simulink library "PoolIir"  (R2022b)
settings: Solver=VariableStepAuto  StartTime=0.0  StopTime=10.0  RelTol=1e-3
undefined symbols (not defined in the file or in its folder): Row
libraries: HandyTextFile x14, TuneVar x5, $bdroot x4, simulink x3, RTC x3, FeaturePath x2, TOP x2, AudioStats x1, CapturedConstLib x1
(part 1 of 2)
settings Model: Creator=sd49596  LastModifiedBy=fz1054048
settings SolverCC: AlgebraicLoopSolver=TrustRegion
settings DebuggingCC: UnconnectedInputMsg=warning  UnconnectedOutputMsg=warning  UnconnectedLineMsg=warning  SFMachineParentedDataDiag=warning  ArithmeticOperatorsInVariantConditions=warning
settings ModelReferenceCC: EnableRefExpFcnMdlSchedulingChecks=on
settings SFSimCC: CustomCodeUndefinedFunction=UseInterfaceOnly
settings RTWCC: DLArmComputeVersion=19.05

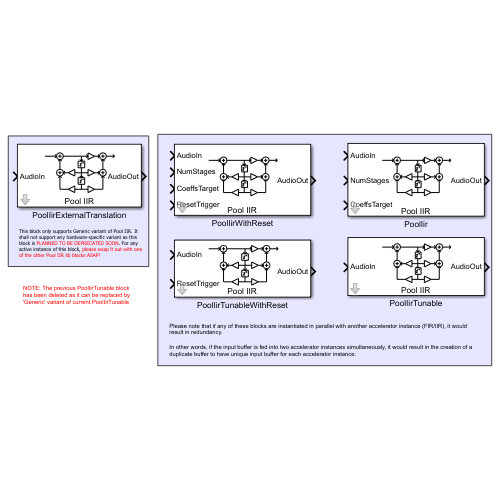
[thumbnail: Simulink's stored preview of the top-level diagram]
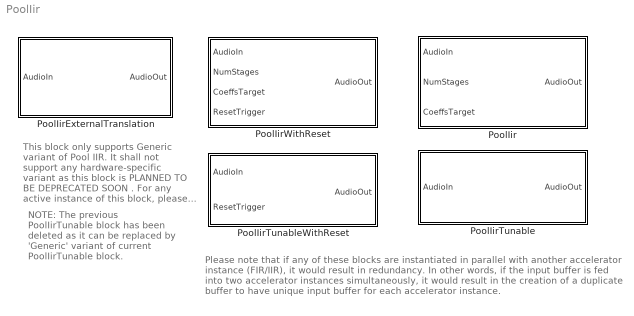
== system PoolIir ==
  note: NOTE: The previous PoolIirTunable block has been deleted as it can be replaced by 'Generic' variant of current PoolIirTunable block.
  note: This block only supports Generic variant of Pool IIR. It shall not support any hardware-specific variant as this block is PLANNED TO BE DEPRECATED SOON . For any active instance of this block, please swap it out with one of the other Pool IIR lib blocks ASAP!
  note: Please note that if any of these blocks are instantiated in parallel with another accelerator instance (FIR/IIR), it would result in redundancy.
      |
      | In other words, if the input buffer is fed into two accelerator instances simultaneously, it would result in the creation of a duplicate buffer to have unique input buffer for each accelerator instance.
  PoolIir : Subsystem  mask(Bose Pool IIR){Config=[]}
      mask prompts: Config "PoolIirConfig"
      mask help:
      | Pool IIR is a configurable multi-channel IIR filter that supports one or more channels. This block only supports the basic signal processing. The number of stages and coefficients need to be passed in in a format expected by the target. The Pool IIR block supports different implementations, which could be configured at build-time:
      |
      | (i)   Generic: IIR filter code not optimized for any processor
      | (ii)  SharcCore: IIR filters executing on core (uses pooliir.asm CRL)
      | (iii) SharcGulAccel: IIR filters executing on IIR hardware accelerator, offloading MIPS usage from core
      | (iv) SharcGxpAccel: IIR filters take advantage of additional accelerators available on GXP processor
      | (v)  Hexagon: TBD
      |
      | NOTE: When using Pool IIR for Sharc-plus based processors, the codeWorkMemory buffer and input buffer should always be mapped to L1 memory to optimize MIPS utilization and avoid audio artifacts.
      mask init:
      | blkh=gcbh;
      | Config=BTConfig.Assert(blkh,Config);
      | 
      | Config.Validate();
      | Config.DoMaskInit(blkh);
      mask Display: DrawPoolIirIcon;
  PoolIirExternalTranslation : Subsystem  InitFcn=warning('''%s'' block will soon be deprecated. Please replace all the active instances of ''PoolIirExternalTranslation'' with an appropriate BTC supported version of Pool IIR located within PoolIir.slx.', gcb);  mask{Config=[], FeatureName=filter}
      mask prompts: Config "PoolIirExternalTranslationConfig"; FeatureName "Feature path name:"
      mask init:
      | blkh=gcbh;
      | Config=BTConfig.Assert(blkh,Config);
      | 
      | BTConfig.InitSetFeatureIfPresent(blkh,'FeatureName');
      | Config.Validate();
      mask Callback Config: BTConfig.CallbackHideIfPresent(gcbh,{'FeatureName'});
      mask TypeOptions FeatureName: FeaturePath/FeatureName
      mask Display: DrawPoolIirIcon;
  PoolIirTunable : Subsystem  mask(Bose Pool IIR Tunable){FeatureName=PoolIirTunableConfig, Config=[]}
      mask prompts: FeatureName "Filter name/purpose"; Config "PoolIirTunableConfig"
      mask help:
      | Pool IIR Tunable is a configurable multi-channel IIR filter that supports one or more channels. This block offers flexibility of tuning the number of stages and coefficients. Different filter coefficients and number of stages (biquads) can be used for each channel filter. The Pool IIR Tunable block supports different implementations, which could be configured at build-time:
      |
      | (i)   Generic: IIR filter code not optimized for any processor
      | (ii)  SharcCore: IIR filters executing on core (uses pooliir.asm CRL)
      | (iii) SharcGulAccel: IIR filters executing on IIR hardware accelerator, offloading MIPS usage from core
      | (iv) SharcGxpAccel: IIR filters take advantage of additional accelerators available on GXP processor
      | (v)  Hexagon: TBD
      |
      | NOTE: When using Pool IIR for Sharc-plus based processors, the codeWorkMemory buffer and input buffer should always be mapped to L1 memory to optimize MIPS utilization and avoid audio artifacts.
      |
      | For more information, please see 'Help'.
      mask init:
      | blkh=gcbh;
      | Config=BTConfig.Assert(blkh,Config);
      | 
      | Config.Validate();
      | Config.DoMaskInit(blkh);
      mask Help:
      | <b>Input signals: </b>
      | AudioIn: input channels [frame size x number of channels]
      | 
      | <b>Output signals: </b>
      | AudioOut: output channels [frame size x number of channels]
      | 
      | <b>Mask parameters: </b>
      | PoolIirTunableConfig
      | Filter name/purpose
      mask TypeOptions FeatureName: PoolIirTunableWithReset/FeatureName
      mask Display: DrawPoolIirIcon;
  PoolIirTunableWithReset : Subsystem  mask(Bose Pool IIR Tunable With Reset){FeatureName=PoolIirTunableConfig, Config=[]}
      mask prompts: FeatureName "Filter name/purpose"; Config "PoolIirTunableWithResetConfig"
      mask help:
      | Pool IIR Tunable is a configurable multi-channel IIR filter that supports one or more channels. This block offers flexibility of tuning the number of stages and coefficients. Different filter coefficients and number of stages (biquads) can be used for each channel filter. The Pool IIR Tunable block supports different implementations, which could be configured at build-time:
      |
      | (i)   Generic: IIR filter code not optimized for any processor
      | (ii)  SharcCore: IIR filters executing on core (uses pooliir.asm CRL)
      | (iii) SharcGulAccel: IIR filters executing on IIR hardware accelerator, offloading MIPS usage from core
      | (iv) SharcGxpAccel: IIR filters take advantage of additional accelerators available on GXP processor
      | (v)  Hexagon: TBD
      |
      | NOTE: When using Pool IIR for Sharc-plus based processors, the codeWorkMemory buffer and input buffer should always be mapped to L1 memory to optimize MIPS utilization and avoid audio artifacts.
      |
      | For more information, please see 'Help'.
      mask init:
      | blkh=gcbh;
      | Config=BTConfig.Assert(blkh,Config);
      | 
      | BTConfig.InitSetFeatureIfPresent(blkh,'FeatureName');
      | Config.Validate();
      | Config.DoMaskInit(blkh);
      mask Help:
      | <b>Input signals: </b>
      | AudioIn: input channels [frame size x number of channels]
      | ResetTrigger: trigger to reset internal state buffer (usually preferred as a post RMDL step)
      | 
      | <b>Output signals: </b>
      | AudioOut: output channels [frame size x number of channels]
      | 
      | <b>Mask parameters: </b>
      | PoolIirTunableWithResetConfig
      | Filter name/purpose
      mask TypeOptions FeatureName: FeaturePath/FeatureName
      mask Callback Config: BTConfig.CallbackHideIfPresent(gcbh,{'FeatureName'});
      mask Display: DrawPoolIirIcon;
  PoolIirWithReset : Subsystem  mask(Bose Pool IIR With Reset){Config=[]}
      mask prompts: Config "PoolIirWithResetConfig"
      mask help:
      | Pool IIR is a configurable multi-channel IIR filter that supports one or more channels. This block only supports the basic signal processing. The number of stages and coefficients need to be passed in in a format expected by the target. The Pool IIR block supports different implementations, which could be configured at build-time:
      |
      | (i)   Generic: IIR filter code not optimized for any processor
      | (ii)  SharcCore: IIR filters executing on core (uses pooliir.asm CRL)
      | (iii) SharcGulAccel: IIR filters executing on IIR hardware accelerator, offloading MIPS usage from core
      | (iv) SharcGxpAccel: IIR filters take advantage of additional accelerators available on GXP processor
      | (v)  Hexagon: TBD
      |
      | NOTE: When using Pool IIR for Sharc-plus based processors, the codeWorkMemory buffer and input buffer should always be mapped to L1 memory to optimize MIPS utilization and avoid audio artifacts.
      mask init:
      | blkh=gcbh;
      | Config=BTConfig.Assert(blkh,Config);
      | 
      | Config.Validate();
      | Config.DoMaskInit(blkh);
      mask Display: DrawPoolIirIcon;

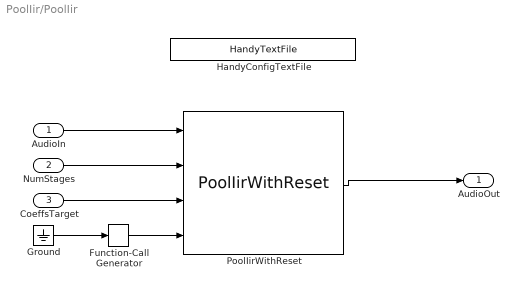
== system PoolIir/PoolIir ==
  AudioIn : Inport
  NumStages : Inport  Port=2
  CoeffsTarget : Inport  Port=3
  Function-Call Generator : simulink/Ports & Subsystems/Function-Call Generator  sample_time=1  numberOfIterations=1  DisallowWideOutput=off  ShowEnablePort=on
  Ground : Ground
  HandyConfigTextFile : HandyTextFile/HandyTextFile  TemplateSource=Config  FileSuffix=File  OpenDialogOnLoad=off  UseThisBlockName=off  AddGrandParentNamePrefix=off  TheDefaultText=% $(FILENAME) $(PREFIX) $(SUFFIX)  ShowInLibBrowser=on
      settings: SourceProductName=Bose Talaria
  PoolIirWithReset : $bdroot/PoolIirWithReset  Config=Config
  AudioOut : Outport
  wires:
  AudioIn/1 -> PoolIirWithReset/1
  PoolIirWithReset/1 -> AudioOut/1
  NumStages/1 -> PoolIirWithReset/2
  CoeffsTarget/1 -> PoolIirWithReset/3
  Function-Call Generator/1 -> PoolIirWithReset/4
  Ground/1 -> Function-Call Generator/1

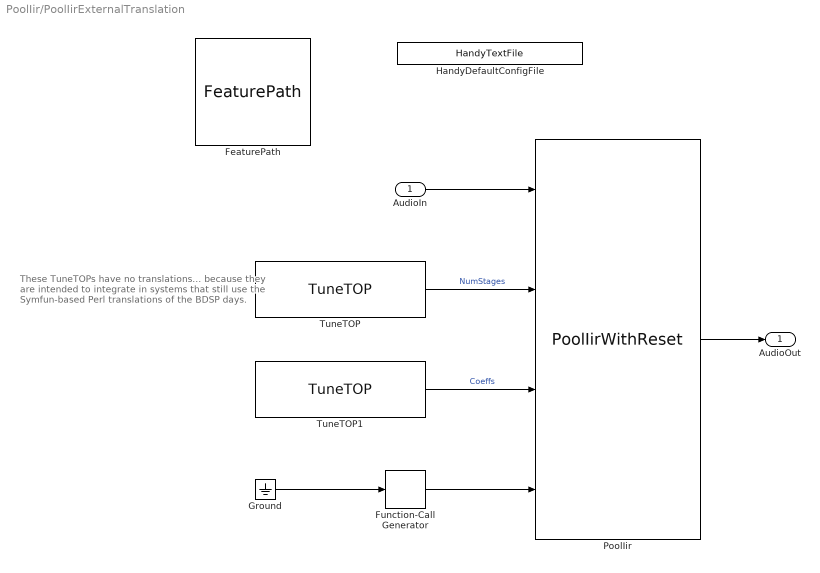
== system PoolIir/PoolIirExternalTranslation ==
  note: These TuneTOPs have no translations... because
      | they are intended to integrate in systems that still
      | use the Symfun-based Perl translations of the
      | BDSP days.
  AudioIn : Inport
  FeaturePath : FeaturePath/FeaturePath  FeatureName=filter  IsGroup=off  GroupNumber=-1  IsModule=off  TriggerInit=[-205 -51 -90 56]
      settings: SourceProductName=Bose Talaria
  Function-Call Generator : simulink/Ports & Subsystems/Function-Call Generator  sample_time=1  numberOfIterations=1  DisallowWideOutput=off  ShowEnablePort=on
  Ground : Ground
  HandyDefaultConfigFile : HandyTextFile/HandyTextFile  TemplateSource=Config  FileSuffix=Init  OpenDialogOnLoad=off  UseThisBlockName=off  AddGrandParentNamePrefix=off  TheDefaultText=|  ShowInLibBrowser=on
      | % $(FILENAME) Setup model parameters for each "Init" callback (e.g. update diagram)
      | sample_rate_in_hertz = 44100;
      | frame_size = 32;
      | sysin_channel_count = 2;
      settings: SourceProductName=Bose Talaria
  PoolIir : $bdroot/PoolIirWithReset  Config=Config.PoolIir
      settings: LibrarySourceBlock=PoolIir/PoolIir
  TuneTOP : TuneVar/TuneTOP  TriggerInit=[-145 172 25 228]  TopName=NumStages  TuneName=NumStages  DataTypeOut=single  TunabilityNumber=1  MinValue=[]  MaxValue=[]  BankNumber=0  PreOverlay=false  PostOverlay=false  UseSameName=on  MaskValue=Config.DefaultNumStages
      settings: SourceProductName=Bose Talaria
  TuneTOP1 : TuneVar/TuneTOP  TriggerInit=[-145 272 25 328]  TopName=Coeffs  TuneName=Coeffs  DataTypeOut=single  TunabilityNumber=1  MinValue=[]  MaxValue=[]  BankNumber=0  PreOverlay=false  PostOverlay=false  UseSameName=on  MaskValue=Config.DefaultSosCoefficients
      settings: SourceProductName=Bose Talaria
  AudioOut : Outport  VectorParamsAs1DForOutWhenUnconnected=off
  wires:
  TuneTOP1/1 -> PoolIir/3  "Coeffs"
  TuneTOP/1 -> PoolIir/2  "NumStages"
  AudioIn/1 -> PoolIir/1
  PoolIir/1 -> AudioOut/1
  Ground/1 -> Function-Call Generator/1
  Function-Call Generator/1 -> PoolIir/4

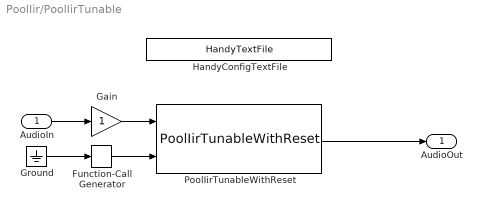
== system PoolIir/PoolIirTunable ==
  AudioIn : Inport
  Function-Call Generator : simulink/Ports & Subsystems/Function-Call Generator  sample_time=1  numberOfIterations=1  DisallowWideOutput=off  ShowEnablePort=on
  Gain : Gain
  Ground : Ground
  HandyConfigTextFile : HandyTextFile/HandyTextFile  TemplateSource=Config  FileSuffix=File  OpenDialogOnLoad=off  UseThisBlockName=off  AddGrandParentNamePrefix=off  TheDefaultText=% $(FILENAME) $(PREFIX) $(SUFFIX)  ShowInLibBrowser=on
      settings: SourceProductName=Bose Talaria
  PoolIirTunableWithReset : $bdroot/PoolIirTunableWithReset  FeatureName=PoolIirTunableConfig  Config=Config
  AudioOut : Outport
  wires:
  AudioIn/1 -> Gain/1
  PoolIirTunableWithReset/1 -> AudioOut/1
  Function-Call Generator/1 -> PoolIirTunableWithReset/2
  Ground/1 -> Function-Call Generator/1
  Gain/1 -> PoolIirTunableWithReset/1

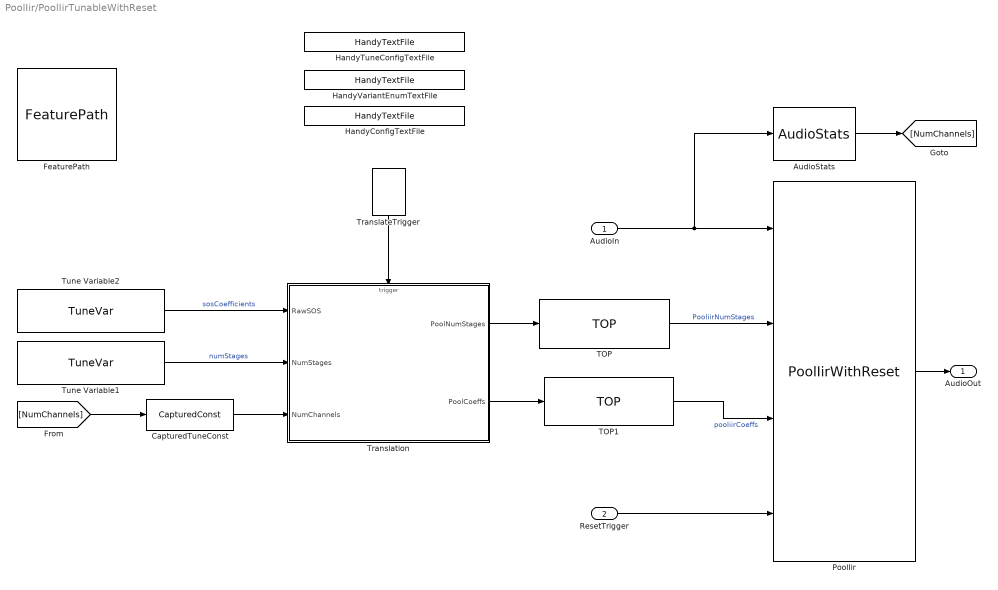
== system PoolIir/PoolIirTunableWithReset ==
  AudioIn : Inport
  ResetTrigger : Inport  Port=2
  AudioStats : AudioStats/AudioStats  DoSampleRate=off  TypeSampleRate=Inherit: auto  DoCallRate=off  TypeCallRate=Inherit: auto  DoFrameSize=off  TypeFrameSize=Inherit: auto  DoChannelCount=on  TypeChannelCount=int32  DoTaskRateFactor=off  TypeTaskRateFactor=Inherit: auto  MacroNameRoot=AUDIO  MacroNameRootEval='AUDIO'  IsMacroNameEval=off  MacroSampleRate=off  MacroCallRate=off  MacroFrameSize=off  MacroChannelCount=off  MacroTaskRateFactor=off  MacroTaskId=off  ValidateSampleRate=off  ValueSampleRate=[]  ValidateCallRate=off  ValueCallRate=[]  ValidateFrameSize=off  ValueFrameSize=[]  ValidateChannelCount=off  ValueChannelCount=[]  ValidateTaskRateFactor=off  ValueTaskRateFactor=[]
      settings: SourceProductName=Bose Talaria
  CapturedTuneConst : CapturedConstLib/CapturedConst  TriggerInit=[-600 302 -500 338]  Role=Automatic
      settings: SourceProductName=Bose Talaria
  FeaturePath : FeaturePath/FeaturePath  FeatureName=PoolIirTunableConfig  IsGroup=off  GroupNumber=-1  IsModule=off  TriggerInit=[-750 -81 -635 26]
      settings: SourceProductName=Bose Talaria
  HandyConfigTextFile : HandyTextFile/HandyTextFile  TemplateSource=Config  FileSuffix=File  OpenDialogOnLoad=off  UseThisBlockName=off  AddGrandParentNamePrefix=off  TheDefaultText=% $(FILENAME) $(PREFIX) $(SUFFIX)  ShowInLibBrowser=on
      settings: SourceProductName=Bose Talaria
  HandyTuneConfigTextFile : HandyTextFile/HandyTextFile  TemplateSource=TuneConfig  FileSuffix=File  OpenDialogOnLoad=off  UseThisBlockName=off  AddGrandParentNamePrefix=off  TheDefaultText=% $(FILENAME) $(PREFIX) $(SUFFIX)  ShowInLibBrowser=on
      settings: SourceProductName=Bose Talaria
  HandyVariantEnumTextFile : HandyTextFile/HandyTextFile  TemplateSource=VariantEnum  FileSuffix=File  OpenDialogOnLoad=off  UseThisBlockName=off  AddGrandParentNamePrefix=off  TheDefaultText=% $(FILENAME) $(PREFIX) $(SUFFIX)  ShowInLibBrowser=on
      settings: SourceProductName=Bose Talaria
  PoolIir : $bdroot/PoolIirWithReset  Config=Config
  TOP : TOP/TOP  TriggerInit=[-145 187 5 243]  TopName=PooliirNumStages  DataTypeOut=uint32  BankNumber=0  PreOverlay=false  PostOverlay=Config.BreedObj.PostOverlayRequired  CompatibilityString=Config.Breed  Role=Automatic
      settings: SourceProductName=Bose Talaria
  TOP1 : TOP/TOP  TriggerInit=[-140 277 10 333]  TopName=pooliirCoeffs  DataTypeOut=single  BankNumber=0  PreOverlay=false  PostOverlay=Config.BreedObj.PostOverlayRequired  CompatibilityString=Config.Breed  Role=Automatic
      settings: SourceProductName=Bose Talaria
  TranslateTrigger : TuneVar/TranslateTrigger  TriggerInit=[-339 35 -301 90]
      settings: SourceProductName=Bose Talaria
  Translation : MATLAB Function  TreatAsAtomicUnit=on  mask{MaxNumStages=Config.MaxNumStages, Breed=Config.Breed}
  Tune Variable1 : TuneVar/TuneVar  TuneName=numStages  SpecifyMaxSize=off  VariableDim=1 (Row)  MaxSize=[1 1]  TunabilityNumber=1  MinValue=[]  MaxValue=[]  TriggerInit=[-750 235 -580 285]  MaskValue=Config.TuneVarNumStages
      settings: SourceProductName=Bose Talaria
  Tune Variable2 : TuneVar/TuneVar  TuneName=sosCoefficients  SpecifyMaxSize=on  VariableDim=1 (Row)  MaxSize=[Config.MaxNumStages 6]  TunabilityNumber=1  MinValue=[]  MaxValue=[]  TriggerInit=[-750 175 -580 225]  MaskValue=Config.TuneVarSosCoefficients
      settings: SourceProductName=Bose Talaria
  AudioOut : Outport  VectorParamsAs1DForOutWhenUnconnected=off
  wires:
  AudioIn/1 -> AudioStats/1, PoolIir/1
  TOP/1 -> PoolIir/2  "PooliirNumStages"
  TOP1/1 -> PoolIir/3  "pooliirCoeffs"
  PoolIir/1 -> AudioOut/1
  TranslateTrigger/1 -> Translation/Trigger
  Tune Variable2/1 -> Translation/1(RawSOS)  "sosCoefficients"
  Translation/2(PoolCoeffs) -> TOP1/1
  Translation/1(PoolNumStages) -> TOP/1
  Tune Variable1/1 -> Translation/2(NumStages)  "numStages"
  ResetTrigger/1 -> PoolIir/4
  AudioStats/1 -> [NumChannels]
  [NumChannels] -> CapturedTuneConst/1
  CapturedTuneConst/1 -> Translation/3(NumChannels)

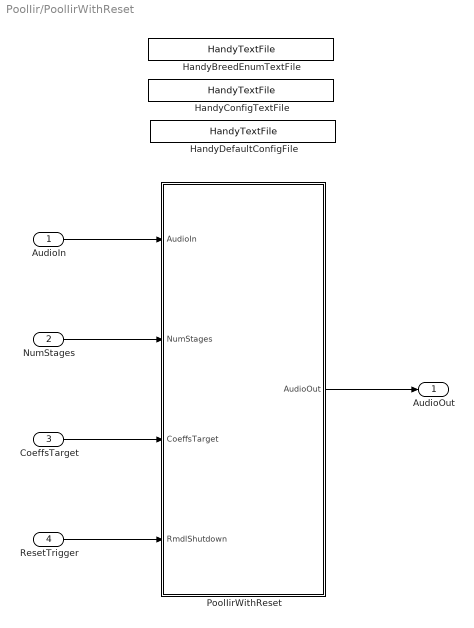
== system PoolIir/PoolIirWithReset ==
  AudioIn : Inport
  NumStages : Inport  Port=2
  CoeffsTarget : Inport  Port=3
  ResetTrigger : Inport  Port=4
  HandyBreedEnumTextFile : HandyTextFile/HandyTextFile  TemplateSource=<dialog fields>  FileSuffix=BreedEnum  OpenDialogOnLoad=off  UseThisBlockName=off  AddGrandParentNamePrefix=off  TheDefaultText=% $(FILENAME) $(PREFIX) $(SUFFIX)  ShowInLibBrowser=on
      settings: SourceProductName=Bose Talaria
  HandyConfigTextFile : HandyTextFile/HandyTextFile  TemplateSource=Config  FileSuffix=File  OpenDialogOnLoad=off  UseThisBlockName=off  AddGrandParentNamePrefix=off  TheDefaultText=% $(FILENAME) $(PREFIX) $(SUFFIX)  ShowInLibBrowser=on
      settings: SourceProductName=Bose Talaria
  HandyDefaultConfigFile : HandyTextFile/HandyTextFile  TemplateSource=Config  FileSuffix=Init  OpenDialogOnLoad=off  UseThisBlockName=off  AddGrandParentNamePrefix=off  TheDefaultText=|  ShowInLibBrowser=on
      | % $(FILENAME) Setup model parameters for each "Init" callback (e.g. update diagram)
      | sample_rate_in_hertz = 44100;
      | frame_size = 32;
      | sysin_channel_count = 2;
      settings: SourceProductName=Bose Talaria
  PoolIirWithReset : Subsystem  Variant=on
  AudioOut : Outport  VectorParamsAs1DForOutWhenUnconnected=off
  wires:
  AudioIn/1 -> PoolIirWithReset/1(AudioIn)
  ResetTrigger/1 -> PoolIirWithReset/4(RmdlShutdown)
  NumStages/1 -> PoolIirWithReset/2(NumStages)
  CoeffsTarget/1 -> PoolIirWithReset/3(CoeffsTarget)
  PoolIirWithReset/1(AudioOut) -> AudioOut/1

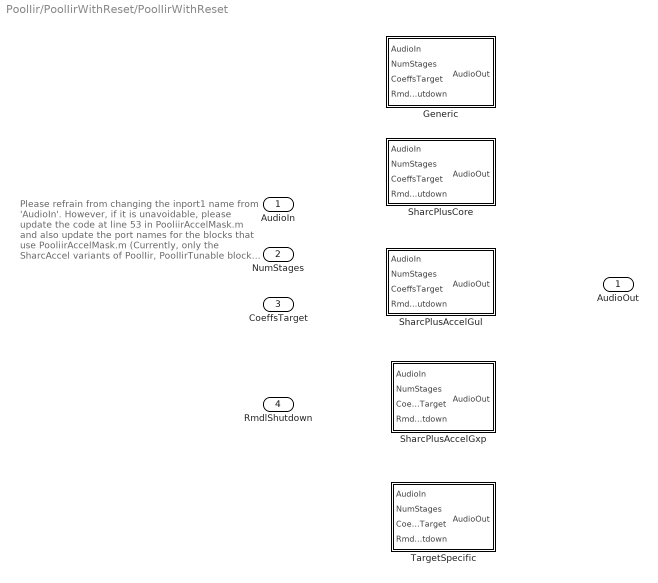
== system PoolIir/PoolIirWithReset/PoolIirWithReset ==
  note: Please refrain from changing the inport1 name from 'AudioIn'. However, if it is unavoidable, please update the code at line 53 in PooliirAccelMask.m and also update the port names for the blocks that use PooliirAccelMask.m (Currently, only the SharcAccel variants of PoolIir, PoolIirTunable block and PooliirAccelRmdl block uses that.)
  AudioIn : Inport
  NumStages : Inport  Port=2
  CoeffsTarget : Inport  Port=3
  RmdlShutdown : Inport  Port=4
  Generic : Subsystem  VariantControl=(default)
  SharcPlusAccelGul : Subsystem  VariantControl=Config.Breed == AsdHwEnum.SharcPlusAccelGul
  SharcPlusAccelGxp : Subsystem  VariantControl=Config.Breed == AsdHwEnum.SharcPlusAccelGxp
  SharcPlusCore : Subsystem  VariantControl=Config.Breed == AsdHwEnum.SharcPlusCore
  TargetSpecific : Subsystem  VariantControl=(Config.Breed == AsdHwEnum.Hexagon) || (Config.Breed == AsdHwEnum.ArmNeonV7V8)
  AudioOut : Outport

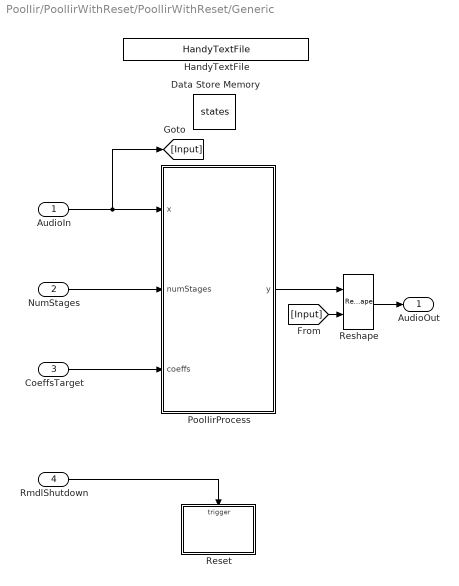
== system PoolIir/PoolIirWithReset/PoolIirWithReset/Generic ==
  AudioIn : Inport
  NumStages : Inport  Port=2
  CoeffsTarget : Inport  Port=3
  RmdlShutdown : Inport  Port=4
  Data Store Memory : DataStoreMemory  DataStoreName=states  InitialValue=Config.BreedObj.CodeWorkMemoryInitVal  ShowAdditionalParam=off  OutDataTypeStr=single
  HandyTextFile : HandyTextFile/HandyTextFile  TemplateSource=<dialog fields>  FileSuffix=BreedEnum  OpenDialogOnLoad=off  UseThisBlockName=off  AddGrandParentNamePrefix=on  TheDefaultText=% $(FILENAME) $(PREFIX) $(SUFFIX)  ShowInLibBrowser=on
      settings: SourceProductName=Bose Talaria
  PoolIirProcess : MATLAB Function  TreatAsAtomicUnit=on
  Reset : MATLAB Function  TreatAsAtomicUnit=on
  Reshape : Reshape  OutputDimensionality=Derive from reference input port
  AudioOut : Outport  VectorParamsAs1DForOutWhenUnconnected=off
  wires:
  RmdlShutdown/1 -> Reset/Trigger
  CoeffsTarget/1 -> PoolIirProcess/3(coeffs)
  NumStages/1 -> PoolIirProcess/2(numStages)
  Reshape/1 -> AudioOut/1
  AudioIn/1 -> [Input], PoolIirProcess/1(x)
  PoolIirProcess/1(y) -> Reshape/1
  [Input] -> Reshape/2

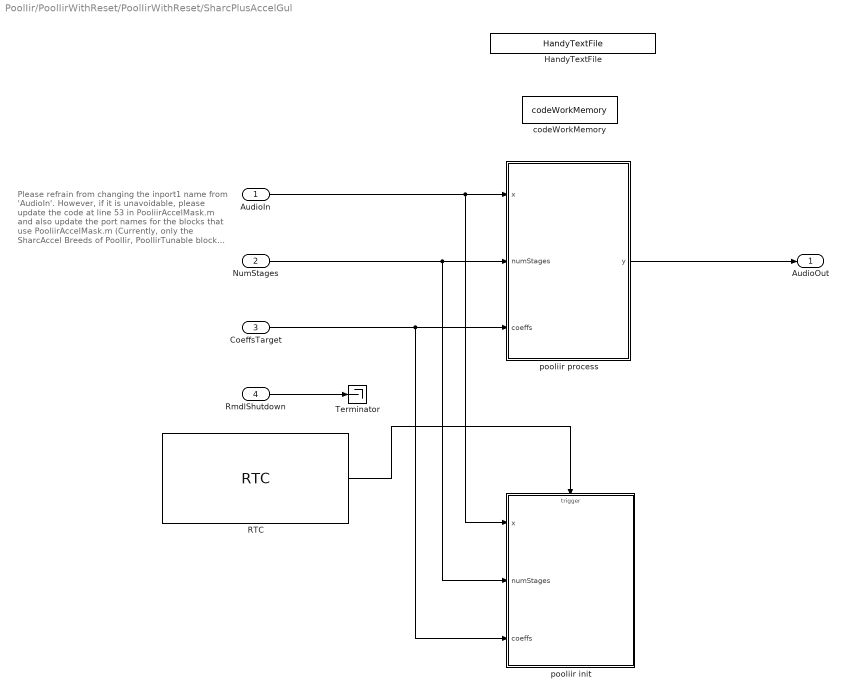
== system PoolIir/PoolIirWithReset/PoolIirWithReset/SharcPlusAccelGul ==
  note: Please refrain from changing the inport1 name from 'AudioIn'. However, if it is unavoidable, please update the code at line 53 in PooliirAccelMask.m and also update the port names for the blocks that use PooliirAccelMask.m (Currently, only the SharcAccel Breeds of PoolIir, PoolIirTunable block and PooliirAccelRmdl block uses that.)
  AudioIn : Inport
  NumStages : Inport  Port=2
  CoeffsTarget : Inport  Port=3
  RmdlShutdown : Inport  Port=4
  HandyTextFile : HandyTextFile/HandyTextFile  TemplateSource=<dialog fields>  FileSuffix=BreedEnum  OpenDialogOnLoad=off  UseThisBlockName=off  AddGrandParentNamePrefix=on  TheDefaultText=% $(FILENAME) $(PREFIX) $(SUFFIX)  ShowInLibBrowser=on
      settings: SourceProductName=Bose Talaria
  RTC : RTC/RTC  REQ_Priority=RTC_Mask.NormalPriority  RequestAtInit=on  EnableRequest=on  REQElemType1=uint32  REQElemWidth1=1  REQElemInitial1=[]  REQElemType2=uint32  REQElemWidth2=1  REQElemInitial2=[]  REQElemType3=uint32  REQElemWidth3=1  REQElemInitial3=[]  REQElemType4=uint32  REQElemWidth4=1  REQElemInitial4=[]  REQElemType5=uint32  REQElemWidth5=1  REQElemInitial5=[]  REQElemType6=uint32  REQElemWidth6=1  REQElemInitial6=[]  REQElemType7=uint32  REQElemWidth7=1  REQElemInitial7=[]  REQElemType8=uint32  REQElemWidth8=1  REQElemInitial8=[]  REQElemType9=uint32  REQElemWidth9=1  REQElemInitial9=[]  REQElemType10=uint32  REQElemWidth10=1  REQElemInitial10=[]  EnableResponse=off  EnableRSP_StatusIn=off  RSPElemType1=uint32  RSPElemWidth1=1  RSPElemType2=uint32  RSPElemWidth2=1  RSPElemType3=uint32  RSPElemWidth3=1  RSPElemType4=uint32  RSPElemWidth4=1  RSPElemType5=uint32  RSPElemWidth5=1  RSPElemType6=uint32  RSPElemWidth6=1  RSPElemType7=uint32  RSPElemWidth7=1  RSPElemType8=uint32  RSPElemWidth8=1  RSPElemType9=uint32  RSPElemWidth9=1  RSPElemType10=uint32  RSPElemWidth10=1  EnableNotification=off  EnableNTF_PrepTrig=off  NTFElemType1=uint32  NTFElemWidth1=1  NTFElemType2=uint32  NTFElemWidth2=1  NTFElemType3=uint32  NTFElemWidth3=1  NTFElemType4=uint32  NTFElemWidth4=1  NTFElemType5=uint32  NTFElemWidth5=1  NTFElemType6=uint32  NTFElemWidth6=1  NTFElemType7=uint32  NTFElemWidth7=1  NTFElemType8=uint32  NTFElemWidth8=1  NTFElemType9=uint32  NTFElemWidth9=1  NTFElemType10=uint32  NTFElemWidth10=1  MaskMessageName=PoolIirSharcPlusAccelGulInitReset
      settings: SourceProductName=Bose Talaria
  Terminator : Terminator
  codeWorkMemory : DataStoreMemory  DataStoreName=codeWorkMemory  WriteAfterWriteMsg=warning  InitialValue=Config.BreedObj.CodeWorkMemoryInitVal  ShowAdditionalParam=off  OutDataTypeStr=single
  pooliir init : MATLAB Function  TreatAsAtomicUnit=on  RTWFcnName=foo
  pooliir process : MATLAB Function  TreatAsAtomicUnit=on
  AudioOut : Outport  VectorParamsAs1DForOutWhenUnconnected=off
  wires:
  RmdlShutdown/1 -> Terminator/1
  CoeffsTarget/1 -> pooliir process/3(coeffs), pooliir init/3(coeffs)
  AudioIn/1 -> pooliir init/1(x), pooliir process/1(x)
  NumStages/1 -> pooliir process/2(numStages), pooliir init/2(numStages)
  RTC/1 -> pooliir init/Trigger
  pooliir process/1(y) -> AudioOut/1

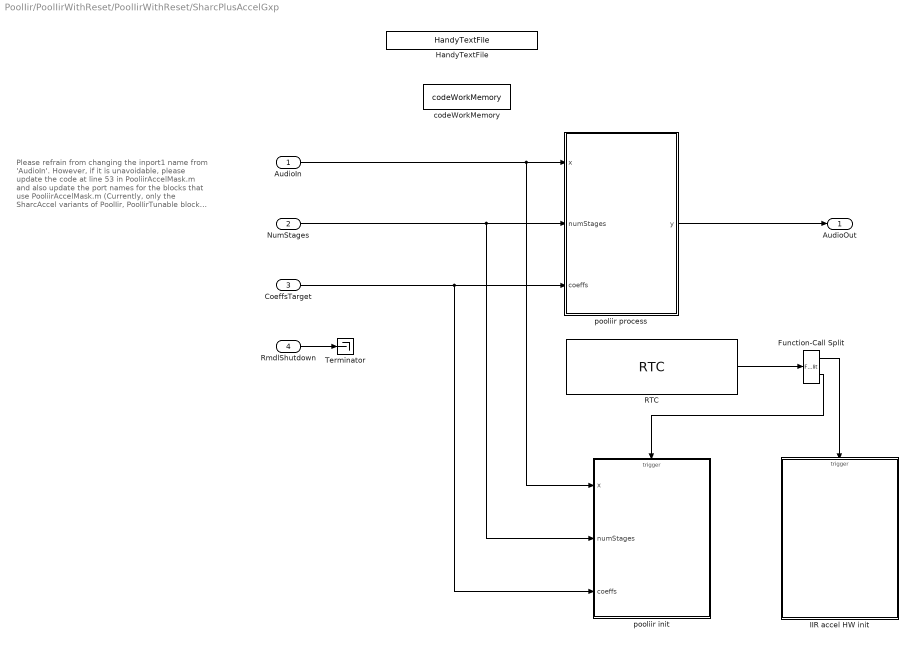
== system PoolIir/PoolIirWithReset/PoolIirWithReset/SharcPlusAccelGxp ==
  note: Please refrain from changing the inport1 name from 'AudioIn'. However, if it is unavoidable, please update the code at line 53 in PooliirAccelMask.m and also update the port names for the blocks that use PooliirAccelMask.m (Currently, only the SharcAccel variants of PoolIir, PoolIirTunable block and PooliirAccelRmdl block uses that.)
  AudioIn : Inport
  NumStages : Inport  Port=2
  CoeffsTarget : Inport  Port=3
  RmdlShutdown : Inport  Port=4
  Function-Call Split : FunctionCallSplit  NumOutputPorts=2  OutputPortLayout=default
  HandyTextFile : HandyTextFile/HandyTextFile  TemplateSource=<dialog fields>  FileSuffix=BreedEnum  OpenDialogOnLoad=off  UseThisBlockName=off  AddGrandParentNamePrefix=on  TheDefaultText=% $(FILENAME) $(PREFIX) $(SUFFIX)  ShowInLibBrowser=on
      settings: SourceProductName=Bose Talaria
  IIR accel HW init : MATLAB Function  TreatAsAtomicUnit=on  RTWFcnName=foo  mask{CoreId=Config.BreedObj.CoreId, AccelDeviceId=Config.BreedObj.AccelDeviceId}
  RTC : RTC/RTC  REQ_Priority=RTC_Mask.NormalPriority  RequestAtInit=on  EnableRequest=on  REQElemType1=uint32  REQElemWidth1=1  REQElemInitial1=[]  REQElemType2=uint32  REQElemWidth2=1  REQElemInitial2=[]  REQElemType3=uint32  REQElemWidth3=1  REQElemInitial3=[]  REQElemType4=uint32  REQElemWidth4=1  REQElemInitial4=[]  REQElemType5=uint32  REQElemWidth5=1  REQElemInitial5=[]  REQElemType6=uint32  REQElemWidth6=1  REQElemInitial6=[]  REQElemType7=uint32  REQElemWidth7=1  REQElemInitial7=[]  REQElemType8=uint32  REQElemWidth8=1  REQElemInitial8=[]  REQElemType9=uint32  REQElemWidth9=1  REQElemInitial9=[]  REQElemType10=uint32  REQElemWidth10=1  REQElemInitial10=[]  EnableResponse=off  EnableRSP_StatusIn=off  RSPElemType1=uint32  RSPElemWidth1=1  RSPElemType2=uint32  RSPElemWidth2=1  RSPElemType3=uint32  RSPElemWidth3=1  RSPElemType4=uint32  RSPElemWidth4=1  RSPElemType5=uint32  RSPElemWidth5=1  RSPElemType6=uint32  RSPElemWidth6=1  RSPElemType7=uint32  RSPElemWidth7=1  RSPElemType8=uint32  RSPElemWidth8=1  RSPElemType9=uint32  RSPElemWidth9=1  RSPElemType10=uint32  RSPElemWidth10=1  EnableNotification=off  EnableNTF_PrepTrig=off  NTFElemType1=uint32  NTFElemWidth1=1  NTFElemType2=uint32  NTFElemWidth2=1  NTFElemType3=uint32  NTFElemWidth3=1  NTFElemType4=uint32  NTFElemWidth4=1  NTFElemType5=uint32  NTFElemWidth5=1  NTFElemType6=uint32  NTFElemWidth6=1  NTFElemType7=uint32  NTFElemWidth7=1  NTFElemType8=uint32  NTFElemWidth8=1  NTFElemType9=uint32  NTFElemWidth9=1  NTFElemType10=uint32  NTFElemWidth10=1  MaskMessageName=PoolIirSharcPlusAccelGxpInitReset
      settings: SourceProductName=Bose Talaria
  Terminator : Terminator
  codeWorkMemory : DataStoreMemory  DataStoreName=codeWorkMemory  WriteAfterWriteMsg=warning  InitialValue=Config.BreedObj.CodeWorkMemoryInitVal  ShowAdditionalParam=off  OutDataTypeStr=single
  pooliir init : MATLAB Function  TreatAsAtomicUnit=on  RTWFcnName=foo  mask{AccelDeviceId=Config.BreedObj.AccelDeviceId}
  pooliir process : MATLAB Function  TreatAsAtomicUnit=on
  AudioOut : Outport
  wires:
  RmdlShutdown/1 -> Terminator/1
  CoeffsTarget/1 -> pooliir init/3(coeffs), pooliir process/3(coeffs)
  pooliir process/1(y) -> AudioOut/1
  AudioIn/1 -> pooliir init/1(x), pooliir process/1(x)
  NumStages/1 -> pooliir init/2(numStages), pooliir process/2(numStages)
  RTC/1 -> Function-Call Split/1
  Function-Call Split/2 -> pooliir init/Trigger
  Function-Call Split/1 -> IIR accel HW init/Trigger

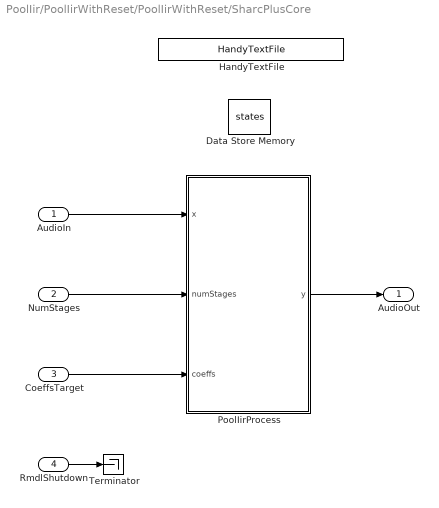
== system PoolIir/PoolIirWithReset/PoolIirWithReset/SharcPlusCore ==
  AudioIn : Inport
  NumStages : Inport  Port=2
  CoeffsTarget : Inport  Port=3
  RmdlShutdown : Inport  Port=4
  Data Store Memory : DataStoreMemory  DataStoreName=states  InitialValue=Config.BreedObj.CodeWorkMemoryInitVal  ShowAdditionalParam=off  OutDataTypeStr=single
  HandyTextFile : HandyTextFile/HandyTextFile  TemplateSource=<dialog fields>  FileSuffix=BreedConfig  OpenDialogOnLoad=off  UseThisBlockName=off  AddGrandParentNamePrefix=on  TheDefaultText=% $(FILENAME) $(PREFIX) $(SUFFIX)  ShowInLibBrowser=on
      settings: SourceProductName=Bose Talaria
  PoolIirProcess : MATLAB Function  TreatAsAtomicUnit=on
  Terminator : Terminator
  AudioOut : Outport  VectorParamsAs1DForOutWhenUnconnected=off
  wires:
  NumStages/1 -> PoolIirProcess/2(numStages)
  PoolIirProcess/1(y) -> AudioOut/1
  AudioIn/1 -> PoolIirProcess/1(x)
  CoeffsTarget/1 -> PoolIirProcess/3(coeffs)
  RmdlShutdown/1 -> Terminator/1

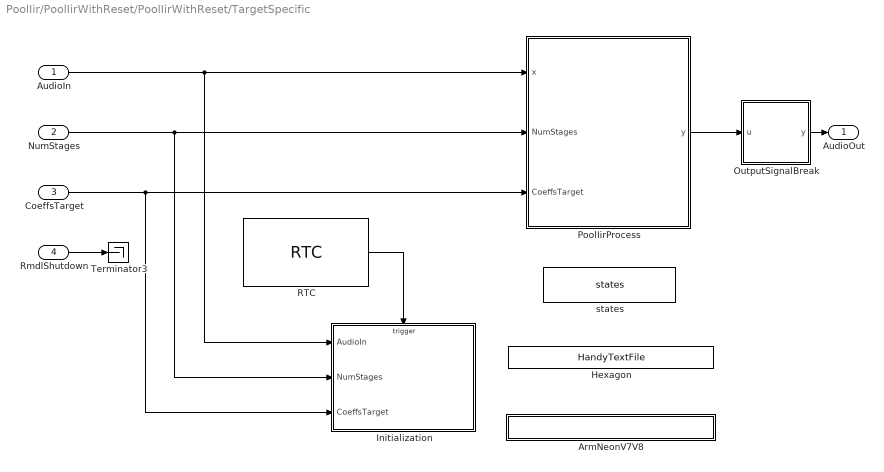
== system PoolIir/PoolIirWithReset/PoolIirWithReset/TargetSpecific ==
  AudioIn : Inport
  NumStages : Inport  Port=2
  CoeffsTarget : Inport  Port=3
  RmdlShutdown : Inport  Port=4
  ArmNeonV7V8 : Subsystem  mask(Talaria Handy Text File){TemplateSource=<dialog fields>, FileSuffix=BreedConfig, OpenDialogOnLoad=off, UseThisBlockName=on, AddGrandParentNamePrefix=on, TheDefaultText=% $(FILENAME) $(PREFIX) $(SUFFIX), ShowInLibBrowser=on}
      mask prompts: TemplateSource "Template Source"; FileSuffix "File suffix:"; OpenDialogOnLoad "Automatically open this dialog if the file is not found when loading the block"; UseThisBlockName "Use *this* block name as file prefix instead of parent subsystem name"; AddGrandParentNamePrefix "Add grandparent subsystem name as additional prefix (ignored if not available)"; TheDefaultText "hidden default text storage:"
      mask help: This block facilitates editing of a text file by opening the file for edit when the block is "opened." If the text file is not found on the path, the opening of this block will display a dialog box enabling the creation of a new file based on a file template.
      settings: OpenFcn=HandyTextFileMask.DoOpenFcn(gcbh);
      mask Help:
      | Advanced settings in the block mask dialog specify settings for the filename and template content.
      | 
      | The Template Source can be set to "dialog fields" to control the filename and defaul content directly from the dialog itself. This mode is self-contained and stores the file template in the block itself. On the downside, since the template is stored in the block, the only way to refresh the template is to open the specific block of interest and edit its internal template.
      | 
      | When Template Source is set to any other value, the handy_template files managed by Talaria are used to create new files. These templates can be refreshed since they are separate template files stored in the filesystem. When these templates are updated, all assocated HandyTextFile blocks use the updated templates when creating new files.
      | 
      | An additional feature for this block is the ability to automatically open this dialog box upon loading of a model. The dialog box is only opened if the automatic open feature is enabled and the file normally opened by the block is not present on the MATLAB path.
      mask TypeOptions TemplateSource: <dialog fields> | Case | Config | Enum | TuneConfig | VariantConfig | VariantEnum
      mask Callback TemplateSource: HandyTextFileMask.CB_TemplateSource(gcbh);
      mask Callback FileSuffix: HandyTextFileMask.CB_FileSuffix(gcbh);
      mask Callback UseThisBlockName: HandyTextFileMask.CB_UseThisBlockName(gcbh);
      mask Callback AddGrandParentNamePrefix: HandyTextFileMask.CB_AddGrandParentNamePrefix(gcbh);
      mask Callback TheDefaultText: HandyTextFileMask.CB_TheDefaultText(gcbh);
      mask DialogControl ButtonCreateFile Prompt: Not on path: C:\Users\fz1054048\AppData\Local\Temp\mwDiff_e01a3046-4e48-40d3-8d4f-d7d319bc3d69\240322134346_79224d29-fc47-4917-b128-1c7ce6418d42\tgt
      mask DialogControl ButtonCreateFile Callback: HandyTextFileMask.CB_CreateFile(gcbh);
      mask DialogControl TextPathWarning Prompt: <html><p style="color:red;text-align:center">Warning: This model is not on the path, so files may not be found.</p></html>
      mask DialogControl AdvancedSettings Prompt: Advanced Block Settings
      mask DialogControl GroupDefaultText Prompt: -------- Default File Content --------
      mask DialogControl TextDefault Prompt: <html><Font color="grey">%&nbsp;PoolIirWithResetArmNeonV7V8VariantConfig.m&nbsp;PoolIirWithResetArmNeonV7V8&nbsp;VariantConfig</Font></html>
      mask DialogControl ButtonEditDefault Prompt: Edit Template File Content
      mask DialogControl ButtonEditDefault Callback: HandyTextFileMask.CB_ButtonEditDefault(gcbh);
      mask DialogControl TextKeywordHelp Prompt: Replacement keywords: $(FILENAME), $(PREFIX), $(SUFFIX)
      mask Display: disp(HandyTextFileMask.GetMaskDisplayText(gcbh));
  Hexagon : HandyTextFile/HandyTextFile  TemplateSource=<dialog fields>  FileSuffix=BreedConfig  OpenDialogOnLoad=off  UseThisBlockName=on  AddGrandParentNamePrefix=on  TheDefaultText=% $(FILENAME) $(PREFIX) $(SUFFIX)  ShowInLibBrowser=on
      settings: SourceProductName=Bose Talaria
  Initialization : Subsystem
  OutputSignalBreak : Subsystem  Variant=on  VariantControl=Choice
  PoolIirProcess : MATLAB Function  TreatAsAtomicUnit=on  mask{Breed=Config.Breed}
  RTC : RTC/RTC  REQ_Priority=RTC_Mask.NormalPriority  RequestAtInit=on  EnableRequest=on  REQElemType1=uint32  REQElemWidth1=1  REQElemInitial1=[]  REQElemType2=uint32  REQElemWidth2=1  REQElemInitial2=[]  REQElemType3=uint32  REQElemWidth3=1  REQElemInitial3=[]  REQElemType4=uint32  REQElemWidth4=1  REQElemInitial4=[]  REQElemType5=uint32  REQElemWidth5=1  REQElemInitial5=[]  REQElemType6=uint32  REQElemWidth6=1  REQElemInitial6=[]  REQElemType7=uint32  REQElemWidth7=1  REQElemInitial7=[]  REQElemType8=uint32  REQElemWidth8=1  REQElemInitial8=[]  REQElemType9=uint32  REQElemWidth9=1  REQElemInitial9=[]  REQElemType10=uint32  REQElemWidth10=1  REQElemInitial10=[]  EnableResponse=off  EnableRSP_StatusIn=off  RSPElemType1=uint32  RSPElemWidth1=1  RSPElemType2=uint32  RSPElemWidth2=1  RSPElemType3=uint32  RSPElemWidth3=1  RSPElemType4=uint32  RSPElemWidth4=1  RSPElemType5=uint32  RSPElemWidth5=1  RSPElemType6=uint32  RSPElemWidth6=1  RSPElemType7=uint32  RSPElemWidth7=1  RSPElemType8=uint32  RSPElemWidth8=1  RSPElemType9=uint32  RSPElemWidth9=1  RSPElemType10=uint32  RSPElemWidth10=1  EnableNotification=off  EnableNTF_PrepTrig=off  NTFElemType1=uint32  NTFElemWidth1=1  NTFElemType2=uint32  NTFElemWidth2=1  NTFElemType3=uint32  NTFElemWidth3=1  NTFElemType4=uint32  NTFElemWidth4=1  NTFElemType5=uint32  NTFElemWidth5=1  NTFElemType6=uint32  NTFElemWidth6=1  NTFElemType7=uint32  NTFElemWidth7=1  NTFElemType8=uint32  NTFElemWidth8=1  NTFElemType9=uint32  NTFElemWidth9=1  NTFElemType10=uint32  NTFElemWidth10=1  MaskMessageName=PoolIirInitReset
      settings: SourceProductName=Bose Talaria
  Terminator3 : Terminator
  states : DataStoreMemory  DataStoreName=states  WriteAfterWriteMsg=warning  InitialValue=Config.BreedObj.DsmStatesInitVal  ShowAdditionalParam=off  OutDataTypeStr=single
  AudioOut : Outport
  wires:
  AudioIn/1 -> PoolIirProcess/1(x), Initialization/1(AudioIn)
  RmdlShutdown/1 -> Terminator3/1
  CoeffsTarget/1 -> PoolIirProcess/3(CoeffsTarget), Initialization/3(CoeffsTarget)
  NumStages/1 -> PoolIirProcess/2(NumStages), Initialization/2(NumStages)
  PoolIirProcess/1(y) -> OutputSignalBreak/1(u)
  OutputSignalBreak/1(y) -> AudioOut/1
  RTC/1 -> Initialization/Trigger

== system PoolIir/PoolIirWithReset/PoolIirWithReset/TargetSpecific/ArmNeonV7V8 ==
  note: Nothing to see here.

== system PoolIir/PoolIirWithReset/PoolIirWithReset/TargetSpecific/Initialization ==
  AudioIn : Inport
  NumStages : Inport  Port=2
  CoeffsTarget : Inport  Port=3
  function : TriggerPort  TriggerType=function-call  VariantControl=(inherit)
  PoolIirInit : MATLAB Function  TreatAsAtomicUnit=on  mask{MaxNumOfThreads=1, MaxNumSosStages=Config.MaxNumStages, Breed=Config.Breed}
  SignalBreak : Subsystem  Variant=on  VariantControl=Choice
  wires:
  AudioIn/1 -> PoolIirInit/1(x)
  SignalBreak/1(y) -> PoolIirInit/3(CoeffsTarget)
  CoeffsTarget/1 -> SignalBreak/1(u)
  NumStages/1 -> PoolIirInit/2(NumStages)

== system PoolIir/PoolIirWithReset/PoolIirWithReset/TargetSpecific/OutputSignalBreak ==
  u : Inport
  ByPass : Subsystem  VariantControl=(default)
  Gain : Subsystem  VariantControl=Config.Breed == AsdHwEnum.Hexagon
  y : Outport

== system PoolIir/PoolIirWithReset/PoolIirWithReset/TargetSpecific/Initialization/SignalBreak ==
  u : Inport
  ByPass : Subsystem  VariantControl=(default)
  SignalBreak : Subsystem  VariantControl=Config.Breed == AsdHwEnum.Hexagon
  y : Outport

== system PoolIir/PoolIirWithReset/PoolIirWithReset/TargetSpecific/OutputSignalBreak/ByPass ==
  u : Inport
  y : Outport
  wires:
  u/1 -> y/1

== system PoolIir/PoolIirWithReset/PoolIirWithReset/TargetSpecific/OutputSignalBreak/Gain ==
  u : Inport
  Gain : Gain
  y : Outport
  wires:
  u/1 -> Gain/1
  Gain/1 -> y/1

== system PoolIir/PoolIirWithReset/PoolIirWithReset/TargetSpecific/Initialization/SignalBreak/ByPass ==
  u : Inport
  y : Outport
  wires:
  u/1 -> y/1

== system PoolIir/PoolIirWithReset/PoolIirWithReset/TargetSpecific/Initialization/SignalBreak/SignalBreak ==
  u : Inport
  SignalBreakFcn : MATLAB Function  TreatAsAtomicUnit=on
  y : Outport
  wires:
  u/1 -> SignalBreakFcn/1(u)
  SignalBreakFcn/1(y) -> y/1

== matlab function PoolIir/PoolIirWithReset/PoolIirWithReset/Generic/Reset ==
  data: states data_store_memory
  events: trigger input FUNCTION_CALL_EVENT
function reset
%#codegen 

% Reset the states DSM to zeros
global states;
states(:) = 0;

== matlab function PoolIir/PoolIirWithReset/PoolIirWithReset/SharcPlusAccelGul/pooliir init ==
  data: x input; numStages input; coeffs input; codeWorkMemory data_store_memory
  events: trigger input FUNCTION_CALL_EVENT
function pooliir_init(x, numStages, coeffs)
% Init function for Pooliir
%
% Parameters:
%   x:              input channels [frame size x number of inputs]
%   numStages:      coefficient sets [total filter lengths x 1]
%   coeffs:         array of filter lengths [number of filters x 1]
%
% Global parameters:
%   codeWorkMemory: working memory set up during roommode reset/init CRL
%                   function call [codeWorkMemorySize x 1]

% Extract configuration information from inputs
[frame_size, num_channels] = size(x);

% Initialize variables
global codeWorkMemory;

% Get the work memory size
workMemorySize = numel(codeWorkMemory);

% Set correct data types
frame_size = uint32(frame_size);
num_channels = uint32(num_channels);
workMemorySize = uint32(workMemorySize);

if(coder.target('MATLAB') || coder.target('Sfun'))
    return; % No init for simulation code
    
else
    % Call the Accel Init function
    y = pooliirAccelInit(x, frame_size, num_channels, numStages, coeffs, ...
        codeWorkMemory, workMemorySize);

    % NOTE: The CRL mechanism requires an output for the function call,
    % and appears to be optimized out if that return value isn't used.
    % This is a dummy operation to make sure CRL ends up in generated code
    codeWorkMemory(1) = y;

end

end


function y = pooliirAccelInit(x, frame_size, num_channels, numStages, coeffs, ...
    workMemory, workMemorySize)
% If target == codegen, error out if no CRL found
coder.replace('-errorifnoreplacement');

% No init simulation code, but need to do something to ensure CRL does not
% get optimized out
y = workMemory(1) + 1;

end

== matlab function PoolIir/PoolIirWithReset/PoolIirWithReset/SharcPlusAccelGul/pooliir process ==
  data: x input; numStages input uint32; y output; coeffs input; codeWorkMemory data_store_memory
function y = pooliir_process(x, numStages, coeffs)
% Process function for Pooliir
%
% Parameters:
%   x:              input channels [frame size x number of inputs]
%   numStages:      coefficient sets [total filter lengths x 1]
%   coeffs:         array of filter lengths [number of filters x 1]
%
% Global parameters:
%   codeWorkMemory: working memory set up during roommode reset/init CRL
%                   function call [codeWorkMemorySize x 1]

% Extract configuration information from inputs
[frame_size, num_channels] = size(x);

% Initialize variables
global codeWorkMemory;

% Set correct data types
frame_size = uint32(frame_size);
num_channels = uint32(num_channels);

% Accelerator selection
if(coder.target('MATLAB') || coder.target('Sfun'))
    % Accelerator simulation
    y = pooliirAccel(x, frame_size, num_channels, numStages, coeffs);
else
    % Accelerator code generation
    y = iir_accelerator_process(x, codeWorkMemory);
end

end

function y = iir_accelerator_process(x, workMemory)
% If target == codegen, error out if no CRL found
coder.replace('-errorifnoreplacement');

[frameSize, numChannels]  = size(x);
y = zeros(frameSize, numChannels, 'single');
end

== matlab function PoolIir/PoolIirWithReset/PoolIirWithReset/SharcPlusCore/PoolIirProcess ==
  data: x input; numStages input uint32; y output single; coeffs input single; states data_store_memory
function y = PooliirProcess(x,numStages, coeffs)
%#codegen

% Parameters:
%   x:              input channels [frame size x number of inputs]
%   numStages:      coefficient sets [total filter lengths x 1]
%   coeffs:         array of filter lengths [number of filters x 1]
%
% Global parameters:
%   states:         State buffer of filter [1x 2*MaxNumStages]
%   RMDLshutdown:   Flag to indicate RMDL is in progress [1 x 1]

% Extract configuration information from inputs
[frame_size, num_channels] = size(x);

% Initialize variables
global states;

% Typecast the variables
frame_size = uint32(frame_size);
num_channels = uint32(num_channels);

% Pooliir Process Selection 
if(coder.target('MATLAB') || coder.target('Sfun'))
    % Simulation
    y = pooliir(x, frame_size, num_channels, numStages, coeffs, states);
else
    % Use assembly CRL for code gen
    y = pooliirCore(x, frame_size, num_channels, numStages, coeffs, states);
end

end

function y = pooliirCore(x, frame_size, num_channels, numStages, coeffs, states)
% If target == codegen, error out if if pooliir.asm is not found
coder.replace('-errorifnoreplacement');

% Dummy code to avoid this function from getting optimized out during code
% gen
[frameSize, numChannels]  = size(x);
y = zeros(frameSize, numChannels, 'single');
end

== matlab function PoolIir/PoolIirWithReset/PoolIirWithReset/TargetSpecific/Initialization/PoolIirInit ==
  data: x input; NumStages input; CoeffsTarget input; states data_store_memory; Breed parameter; MaxNumOfThreads parameter; MaxNumSosStages parameter
function PoolIirInit(x, NumStages, CoeffsTarget, Breed, MaxNumOfThreads, MaxNumSosStages)
% Process function for Pooliir
%
% Parameters:
%   x:                  input channels [frame size x number of inputs]
%   NumStages:          array of filter lengths [NumChannels x 1]
%   CoeffsTarget:       coefficient sets [total filter lengths x 1]
%
% Global parameters:
%   states:             working memory set up during roommode reset/init CRL
%                       function call [StatesSize x 1]
%--------------------------------------------------------------------------

% Extract configuration information from inputs
[FrameSize, NumChannels] = size(x);

% Initialize variables
global states;

% Get the work memory size
StatesSize = numel(states);


if(coder.target('MATLAB') || coder.target('Sfun'))

else
    switch(Breed)
        case{AsdHwEnum.Hexagon}
             NumCoeffPerSosStage = 4;
             y = pooliir_hexagon_init(single(x), uint32(FrameSize), uint32(NumChannels), uint32(NumStages), single(CoeffsTarget), ...
                                     single(states), uint32(StatesSize),uint32(MaxNumOfThreads), uint32(MaxNumSosStages*NumCoeffPerSosStage));
             states(1) = y; 

        case{AsdHwEnum.ArmNeonV7V8}
            y = pooliir_armv7v8_init(single(x), uint32(FrameSize), uint32(NumChannels), uint32(NumStages), single(CoeffsTarget), ...
                                 single(states), uint32(StatesSize));
            % NOTE: The CRL mechanism requires an output for the function call,
            % and appears to be optimized out if that return value isn't used. 
            % This is a dummy operation to make sure CRL ends up in generated code
            states(1) = y; 
        otherwise
            error('Invalid Breed type: [%s]', string(Breed));
    end
end
end


function y = pooliir_hexagon_init(x, frame_size, num_channels, numStages, coeffs, ...
                              states, StatesSize,numThreads,MaxNumSosCoeff)
% If target == codegen, error out if no CRL found
coder.replace('-errorifnoreplacement');

% No init simulation code, but need to do something to ensure CRL does not
% get optimized out
y = states(1) + 1;

end


function y = pooliir_armv7v8_init(x, frame_size, num_channels, numStages, coeffs, ...
                              states, StatesSize)
% If target == codegen, error out if no CRL found
coder.replace('-errorifnoreplacement');

% No init simulation code, but need to do something to ensure CRL does not
% get optimized out
y = states(1) + 1;

end

== matlab function PoolIir/PoolIirWithReset/PoolIirWithReset/TargetSpecific/PoolIirProcess ==
  data: x input; y output; NumStages input; CoeffsTarget input; states data_store_memory; Breed parameter
function y = PoolIirProcess(x, NumStages, CoeffsTarget, Breed)
% Process function for Pooliir
%
% Parameters:
%   x:              input channels [frame size x number of inputs]
%   NumStages:      array of filter lengths per channel [NumChannels x 1]
%   CoeffsTarget:   coefficient set used for the specific target [total sim filter lengths x 1]
% 
% Global parameters:
%   states: working memory set up during roommode reset/init CRL
%                   function call [StatesSize x 1]
%--------------------------------------------------------------------------

% Extract configuration information from inputs
[~, NumChannels] = size(x);

% Initialize variables
global states;
        
if(coder.target('MATLAB') || coder.target('Sfun'))
    switch(Breed)
        case{AsdHwEnum.Hexagon}
            y = PoolIirHexagonSimFcn(single(x), uint32(NumChannels), uint32(NumStages), single(CoeffsTarget), uint32(states));
        case{AsdHwEnum.ArmNeonV7V8}
            y = PoolIirArmNeonV7V8SimFcn(single(x), uint32(NumChannels), uint32(NumStages), single(CoeffsTarget), uint32(states));
    end
else
    switch(Breed)
        case{AsdHwEnum.Hexagon}
            y = pooliir_hexagon_process(single(x), single(states));
        case{AsdHwEnum.ArmNeonV7V8}
            y = pooliir_armv7v8_process(single(x), single(states));
    end
end
end

function y = pooliir_hexagon_process(x, states)
% If target == codegen, error out if no CRL found
coder.replace('-errorifnoreplacement');

y = zeros(size(x), 'single');
end

function y = pooliir_armv7v8_process(x, states)
% If target == codegen, error out if no CRL found
coder.replace('-errorifnoreplacement');

y = zeros(size(x), 'single');
end

== matlab function PoolIir/PoolIirWithReset/PoolIirWithReset/TargetSpecific/Initialization/SignalBreak/SignalBreak/SignalBreakFcn ==
  data: u input; y output
function y = fcn(u)

y = u;

== matlab function PoolIir/PoolIirTunableWithReset/Translation ==
  data: RawSOS input; NumStages input; PoolNumStages output; PoolCoeffs output; MaxNumStages parameter; Breed parameter; NumChannels input
  events: trigger input FUNCTION_CALL_EVENT
function [PoolNumStages, PoolCoeffs] = pooliirTranslation(RawSOS, NumStages, MaxNumStages, Breed,  NumChannels)
%#codegen

% Translation from raw SOS for pool SOS

% Some build time sanity size checking before calling the translation
if numel(NumStages.Value) ~= NumChannels
    error('Size of num stages has to match number of input channels')
end

if RawSOS.Size(2) ~= 6
    error ('Coefficient pool matrix must have 6 columns')
end

[PoolNumStages, PoolCoeffs] = poolIirTranslation(RawSOS, NumStages, MaxNumStages, Breed);

% VariantStr = char(VariantUint8);
% switch (VariantStr)
%     case {"Generic","SharcPlusCore"}
%         % These variants order biquad coefficients in a compacted form
%         [PoolNumStages, PoolCoeffs] = pooliirTranslationFcn(RawSOS, NumStages, MaxNumStages);
%     case {"SharcPlusAccelGul","SharcPlusAccelGxp"}
%         % These variants order biquad coefficients for the ADI accelerator
%         [PoolNumStages, PoolCoeffs] = pooliirAccelTranslationFcn(RawSOS, NumStages, MaxNumStages);
%     case{"Hexagon"}
%         % Hexagon specific order for biquad coefficients 
%         [PoolNumStages, PoolCoeffs] = PoolIirHexagonTranslationFcn(RawSOS, NumStages, MaxNumStages);
%     case{"ArmNeonV7V8"}
%         [PoolNumStages, PoolCoeffs] = PoolIirArmNeonV7V8TranslationFcn(RawSOS, NumStages, MaxNumStages);
%     otherwise
%         % This is a build-time error, not a translation error. The
%         % selected build-time variant is not supported for translation
%         error('Invalid implementation type: [%s]', VariantStr);
% end

end

== matlab function PoolIir/PoolIirWithReset/PoolIirWithReset/SharcPlusAccelGxp/IIR accel HW init ==
  data: codeWorkMemory data_store_memory; CoreId parameter; AccelDeviceId parameter
  events: trigger input FUNCTION_CALL_EVENT
function iir_accel_hw_init(CoreId, AccelDeviceId)
%[Param:CoreId]
%[Param:AccelDeviceId]

% IIR accelerator one-time initialization of accelerator device
%
% Parameters:
%   accelDeviceId:  Device ID of accelerator to initialize (scalar)
%   coreId:         DSP core ID accelerator is assigned to (scalar)
%
% Global parameters:
%   codeWorkMemory: working memory set up during roommode reset/init CRL
%                   function call [codeWorkMemorySize x 1]

global codeWorkMemory;

% Set correct data types (note - types already correct in BTC class)
AccelDeviceId = uint32(AccelDeviceId);
CoreId = uint32(CoreId);
    
% Only initialize the accelerator hardware for the accelerator 
% implementation 
if(~coder.target('MATLAB') && ~coder.target('Sfun')) 
    % Code Generation
    % Initialize the accelerator device hardware
    y = iir_accelerator_hw_init(AccelDeviceId, CoreId);
            
    % NOTE: The CRL mechanism requires an output for the function call,
    % and appears to be optimized out if that return value isn't used. 
    % This is a dummy operation to make sure CRL ends up in generated code
    codeWorkMemory(1) = y;
  
end

end


function y = iir_accelerator_hw_init(accelDeviceId, coreId)                         
% If target == codegen, error out if no CRL found
coder.replace('-errorifnoreplacement');

% No init simulation code, but need to do something to ensure CRL does not
% get optimized out
y = coreId + uint32(1);

end
